simulink subsystem "LQR_controller"  (R2022b)
settings: Solver=VariableStepAuto  StartTime=0.0  StopTime=10.0  RelTol=1e-3
model mask{Kx=0, Ke=0}
  mask prompts: Kx "Kx - State Feedback Gain:"; Ke "Ke - Error Gain:"
settings Model: Creator=gotta  LastModifiedBy=gotta

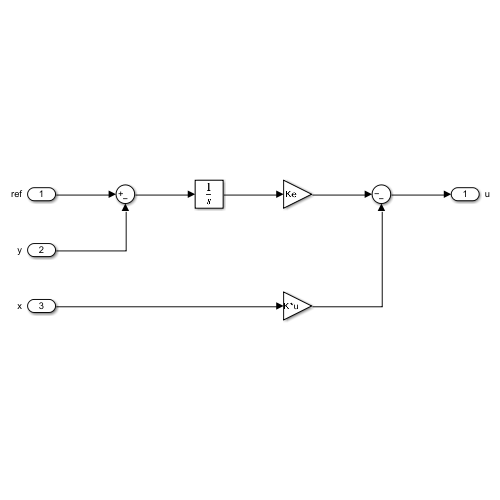
[thumbnail: Simulink's stored preview of the top-level diagram]
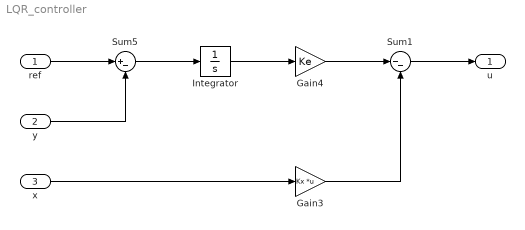
== system LQR_controller ==
  ref : Inport
  y : Inport  Port=2
  x : Inport  Port=3
  Gain3 : Gain  Gain=Kx  Multiplication=Matrix(K*u)
  Gain4 : Gain  Gain=Ke
  Integrator : Integrator
  Sum1 : Sum  Inputs=|--
  Sum5 : Sum  Inputs=|+-
  u : Outport
  wires:
  ref/1 -> Sum5/1
  y/1 -> Sum5/2
  Integrator/1 -> Gain4/1
  Sum5/1 -> Integrator/1
  Gain4/1 -> Sum1/1
  x/1 -> Gain3/1
  Gain3/1 -> Sum1/2
  Sum1/1 -> u/1
